simulink model "air_density_verified"  (R2021b)
settings: Solver=VariableStepAuto  StartTime=0.0  StopTime=500  RelTol=1e-3
undefined symbols (not defined in the file or in its folder): HDBK, MIL, STD
libraries: aerolibatmos2 x4, simulink x1
settings Model: Creator=zhongyuliang  LastModifiedBy=zhongyuliang

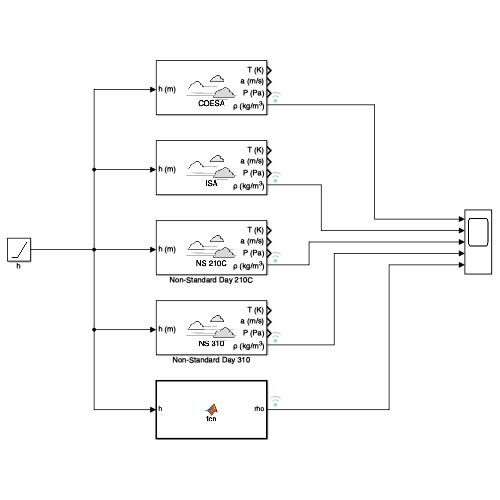
[thumbnail: Simulink's stored preview of the top-level diagram]
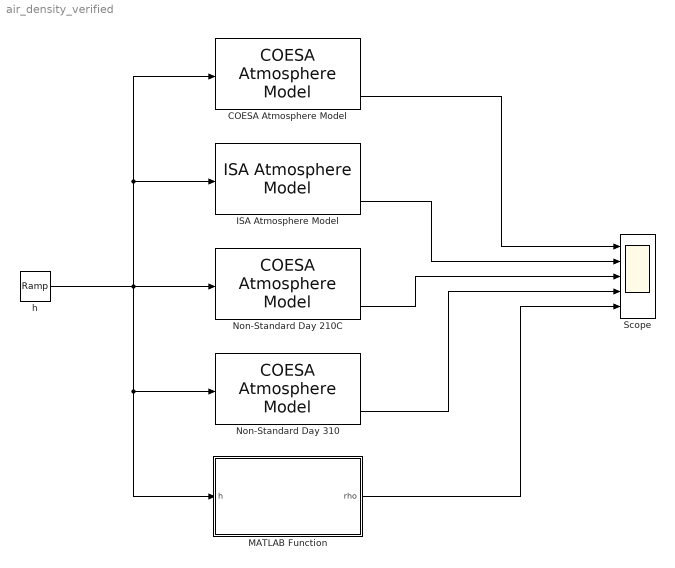
== system air_density_verified ==
  COESA Atmosphere Model : aerolibatmos2/COESA Atmosphere Model  units=Metric (MKS)  spec=1976 COESA-extended U.S. Standard Atmosphere  model=Profile  profile_var=High temperature  profile_percent=1%  profile_alt=5 km (16404 ft)  envelope_var=High temperature  envelope_percent=1%  action=Warning
  ISA Atmosphere Model : aerolibatmos2/ISA Atmosphere Model  custom=off  g=9.80665  gamma=1.4  R=287.0531  L=0.0065  h_trop=11000  h_strat=20000  rho0=1.225  P0=101325  T0=288.15  h0=0
  MATLAB Function : MATLAB Function  TreatAsAtomicUnit=on
  Non-Standard Day 210C : aerolibatmos2/COESA Atmosphere Model  units=Metric (MKS)  spec=MIL-STD-210C  model=Profile  profile_var=High temperature  profile_percent=1%  profile_alt=5 km (16404 ft)  envelope_var=High temperature  envelope_percent=1%  action=Warning
  Non-Standard Day 310 : aerolibatmos2/COESA Atmosphere Model  units=Metric (MKS)  spec=MIL-HDBK-310  model=Profile  profile_var=High temperature  profile_percent=1%  profile_alt=5 km (16404 ft)  envelope_var=High temperature  envelope_percent=1%  action=Warning
  Scope : Scope  NumInputPorts=5
  h : simulink/Sources/Ramp  slope=1  start=0  InitialOutput=0
  wires:
  Non-Standard Day 210C/4 -> Scope/3
  COESA Atmosphere Model/4 -> Scope/1
  ISA Atmosphere Model/4 -> Scope/2
  Non-Standard Day 310/4 -> Scope/4
  MATLAB Function/1(rho) -> Scope/5
  h/1 -> ISA Atmosphere Model/1, COESA Atmosphere Model/1, MATLAB Function/1(h), Non-Standard Day 310/1, Non-Standard Day 210C/1

== matlab function air_density_verified/MATLAB Function ==
  data: h input; rho output
function rho = fcn(h)
    c_h = 1.225;
    c_z = 2.256e-5;
    c_e = 4.2559;
    rho = c_h*(1 - h*c_z)^(c_e);
end
